simulink model "forced_choice"  (Simulink 8.5)
settings: Solver=FixedStepDiscrete  StartTime=0.0  StopTime=Inf  FixedStep=.001  RelTol=1e-3
libraries: limblab x14, slrtlib x2, IntelSMIlibR2007b x1
CloseFcn:
  | rtwprivate ssgencode ModelCloseRequest rwalk_multi_local_v1
settings Model: Creator=limblab  LastModifiedBy=limblab  ExtModeArmWhenConnect=off
settings SolverCC: EnableConcurrentExecution=on
settings DataIOCC: LimitDataPoints=off  SaveFormat=StructureWithTime  SaveState=on  SignalLoggingName=sigsOut
settings OptimizationCC: BlockReduction=off  BooleanDataType=off  OptimizeBlockIOStorage=off  BufferReuse=off  GlobalBufferReuse=off  ExpressionFolding=off  LocalBlockOutputs=off  InitFltsAndDblsToZero=on
settings DebuggingCC: SaveWithParameterizedLinksMsg=none  SignalResolutionControl=TryResolveAllWithWarning  MultiTaskDSMMsg=warning  MultiTaskCondExecSysMsg=none  FcnCallInpInsideContextMsg=UseLocalSettings
settings HardwareCC: ProdIntDivRoundTo=Zero  ProdEndianess=LittleEndian  ProdLongLongMode=on  ProdHWDeviceType=Generic->32-bit x86 compatible  TargetIntDivRoundTo=Floor  TargetEndianess=LittleEndian  TargetHWDeviceType=32-bit xPC Target (Intel Pentium)
settings SFSimCC: SimParseCustomCode=off
settings RTWCC: SystemTargetFile=slrt.tlc  TemplateMakefile=slrt_default_tmf  Description=Simulink Real-Time  GenerateReport=on  RTWCompilerOptimization=on
settings SimulinkRealTimeCC: TargetFcnLib=ansi_tfl_tmw.mat  GeneratePreprocessorConditionals=Disable all

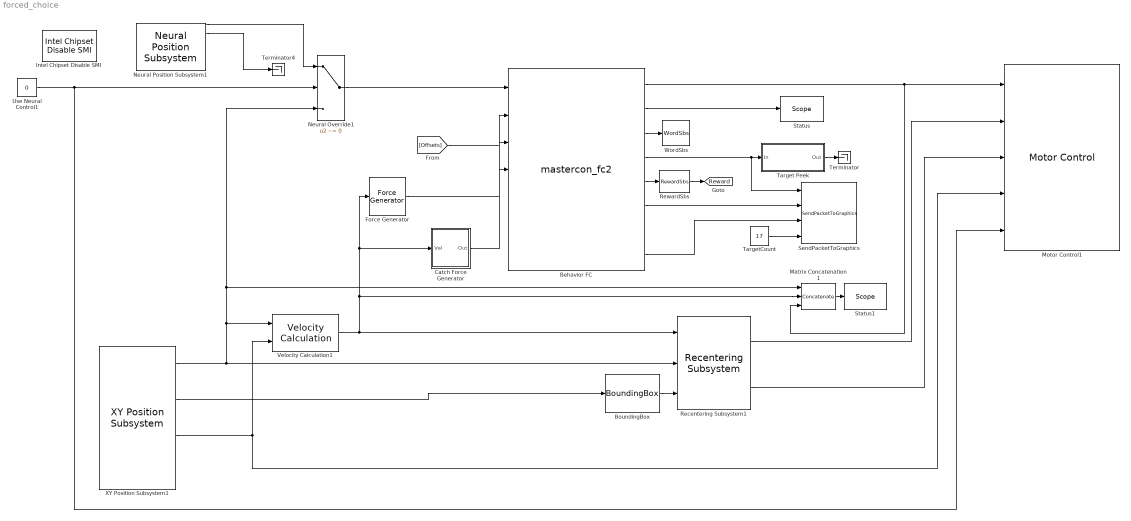
== system forced_choice ==
  Behavior FC : S-Function  FunctionName=mastercon_fc2  Parameters=0 0 3 8 0 0 0 1 0 0 2 .15 .2 .1 .3 .2 .7 .5 1 .2 1 1 1 0 16 .3 1 1
      mask Display:
      | disp('Master Control')
      | port_label('input',1,'pos')
      | port_label('input',2,'pos offsets')
      | port_label('input',3,'force')
      | port_label('input',4,'catch force')
      | port_label('output',1,'force')
      | port_label('output',2,'status')
      | port_label('output',3,'word')
      | port_label('output',4,'targets')
      | port_label('output',5,'reward')
      | port_label('output',6,'tone')
      | port_label('output',7,'version')
      | port_label('output',8,'pos')
  BoundingBox : limblab/BoundingBox
  Catch Force Generator : Subsystem
  Force Generator : limblab/Force Generator
  Intel Chipset Disable SMI : IntelSMIlibR2007b/Intel Chipset Disable SMI
  Matrix Concatenation1 : Concatenate  NumInputs=3
  Motor Control1 : limblab/Motor Control
  Neural Override1 : Switch  Criteria=u2 ~= 0  ZeroCross=off
  Neural Position Subsystem1 : limblab/Neural Position Subsystem
  Recentering Subsystem1 : limblab/Recentering Subsystem
  RewardSbs : limblab/RewardSbs
  SendPacketToGraphics : limblab/SendPacketToGraphics
  Status : slrtlib/Displays and Logging/Scope   scopeno=1  scopetype=Target  autostart=on  viewmode=Numerical  formatstr='%6.0f state,%6.0f rewards,%6.0f aborts,%6.0f fails,%6.0f incompl'  grid=on  ylimits=[-10,10]  nosamples=10  noprepostsamples=0  interleave=10  triggermode=FreeRun  triggersignal=1  trigsignalfromport=off  triggerlevel=0.0  triggerslope=Either  triggerscope=1  triggersample=0  filename=data.dat  mode=Lazy  writesize=512  autorestart=off  dynamicfilemode=off  maxwritefilesize=512*1024^2
  Status1 : slrtlib/Displays and Logging/Scope   scopeno=3  scopetype=Target  autostart=on  viewmode=Numerical  formatstr='%6.0f x,%6.0f y,%6.0f vx,%6.0f vy,%6.0f fx,%6.0f fy'  grid=on  ylimits=[-10,10]  nosamples=10  noprepostsamples=0  interleave=10  triggermode=FreeRun  triggersignal=1  trigsignalfromport=off  triggerlevel=0.0  triggerslope=Either  triggerscope=1  triggersample=0  filename=data.dat  mode=Lazy  writesize=512  autorestart=off  dynamicfilemode=off  maxwritefilesize=512*1024^2
  Target Peek : Subsystem
  TargetCount : Constant  Value=17
  Terminator : Terminator
  Terminator4 : Terminator
  Use Neural Control1 : Constant  Value=0
  Velocity Calculation1 : limblab/Velocity Calculation
  WordSbs : limblab/WordSbs
  XY Position Subsystem1 : limblab/XY Position Subsystem
  tag scope: Reward=global
  wires:
  Velocity Calculation1/1 -> Recentering Subsystem1/1, Force Generator/1, Catch Force Generator/1(Vel), Matrix Concatenation1/2
  XY Position Subsystem1/1 -> Neural Override1/3, Matrix Concatenation1/1, Velocity Calculation1/1, Recentering Subsystem1/2
  Behavior FC/2 -> Status/1
  Behavior FC/3 -> WordSbs/1
  Behavior FC/4 -> Target Peek/1(In), SendPacketToGraphics/1
  Behavior FC/5 -> RewardSbs/1
  BoundingBox/1 -> Recentering Subsystem1/3
  XY Position Subsystem1/3 -> Velocity Calculation1/2, Motor Control1/4
  XY Position Subsystem1/2 -> BoundingBox/1
  Recentering Subsystem1/2 -> Motor Control1/3
  Recentering Subsystem1/1 -> Motor Control1/2
  Behavior FC/8 -> SendPacketToGraphics/3
  Behavior FC/6 -> SendPacketToGraphics/2
  RewardSbs/1 -> [Reward]
  Use Neural Control1/1 -> Motor Control1/5, Neural Override1/2
  Neural Position Subsystem1/1 -> Neural Override1/1
  Neural Position Subsystem1/2 -> Terminator4/1
  Neural Override1/1 -> Behavior FC/1
  Target Peek/1(Out) -> Terminator/1
  TargetCount/1 -> SendPacketToGraphics/4
  Catch Force Generator/1(Out) -> Behavior FC/4
  Force Generator/1 -> Behavior FC/3
  [Offsets] -> Behavior FC/2
  Matrix Concatenation1/1 -> Status1/1
  Behavior FC/1 -> Matrix Concatenation1/3, Motor Control1/1

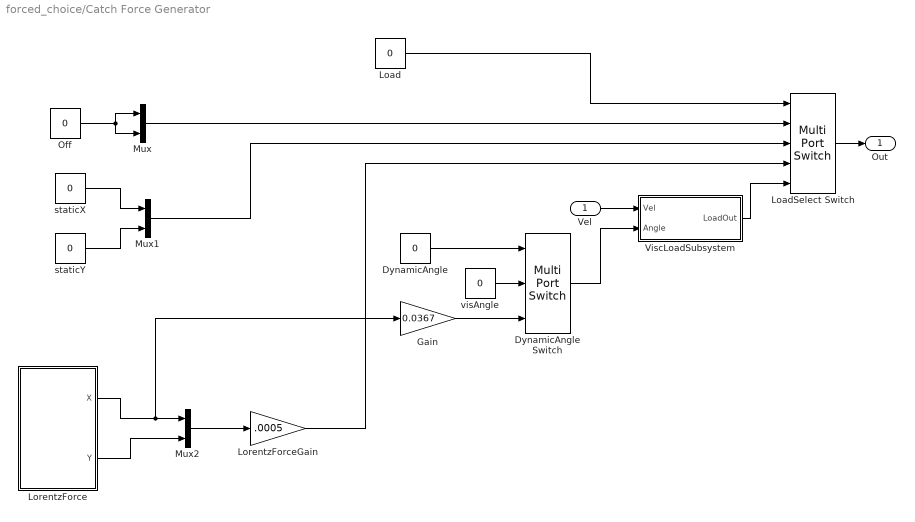
== system forced_choice/Catch Force Generator ==
  Vel : Inport
  DynamicAngle : Constant  Value=0
  DynamicAngle Switch : MultiPortSwitch  DataPortOrder=Zero-based contiguous  Inputs=2  zeroidx=on
  Gain : Gain  Gain=0.0367
  Load : Constant  Value=0
  LoadSelect Switch : MultiPortSwitch  DataPortOrder=Zero-based contiguous  Inputs=4  zeroidx=on
  LorentzForce : Subsystem
  LorentzForceGain : Gain  Gain=.0005
  Mux : Mux  Inputs=2
  Mux1 : Mux  Inputs=2
  Mux2 : Mux  Inputs=2
  Off : Constant  Value=0
  ViscLoadSubsystem : Subsystem
  staticX : Constant  Value=0
  staticY : Constant  Value=0
  visAngle : Constant  Value=0
  Out : Outport
  wires:
  Off/1 -> Mux/2, Mux/1
  LoadSelect Switch/1 -> Out/1
  Mux/1 -> LoadSelect Switch/2
  Load/1 -> LoadSelect Switch/1
  Mux1/1 -> LoadSelect Switch/3
  staticX/1 -> Mux1/1
  staticY/1 -> Mux1/2
  LorentzForce/1(X) -> Mux2/1, Gain/1
  LorentzForce/2(Y) -> Mux2/2
  Mux2/1 -> LorentzForceGain/1
  LorentzForceGain/1 -> LoadSelect Switch/4
  Vel/1 -> ViscLoadSubsystem/1(Vel)
  ViscLoadSubsystem/1(LoadOut) -> LoadSelect Switch/5
  visAngle/1 -> DynamicAngle Switch/2
  DynamicAngle/1 -> DynamicAngle Switch/1
  DynamicAngle Switch/1 -> ViscLoadSubsystem/2(Angle)
  Gain/1 -> DynamicAngle Switch/3

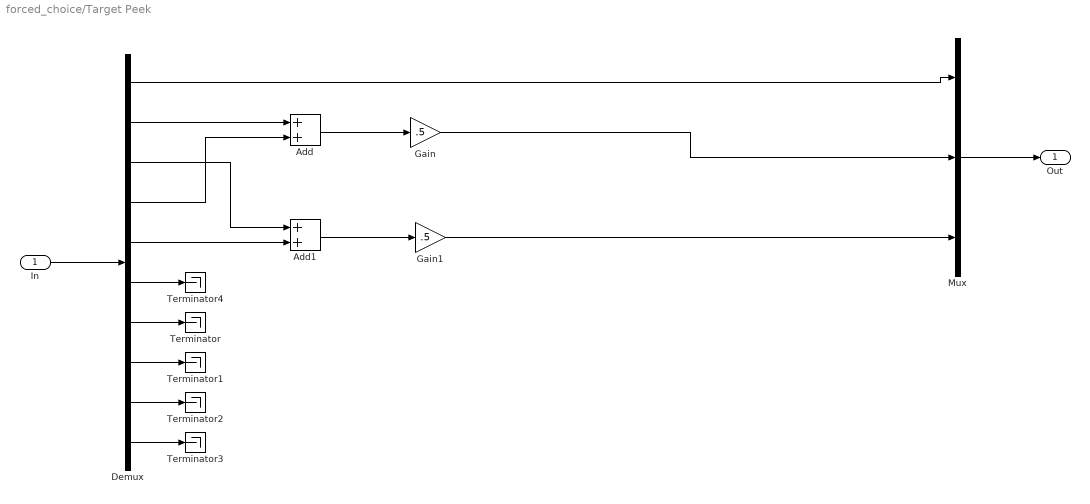
== system forced_choice/Target Peek ==
  In : Inport
  Add : Sum
  Add1 : Sum
  Demux : Demux  Outputs=10
  Gain : Gain  Gain=.5
  Gain1 : Gain  Gain=.5
  Mux : Mux  Inputs=3
  Terminator{,1..4} (5 alike) : Terminator
  Out : Outport
  wires:
  In/1 -> Demux/1
  Mux/1 -> Out/1
  Demux/1 -> Mux/1
  Add/1 -> Gain/1
  Add1/1 -> Gain1/1
  Gain1/1 -> Mux/3
  Demux/7 -> Terminator/1
  Demux/8 -> Terminator1/1
  Demux/9 -> Terminator2/1
  Demux/10 -> Terminator3/1
  Demux/2 -> Add/1
  Demux/4 -> Add/2
  Demux/3 -> Add1/1
  Demux/5 -> Add1/2
  Demux/6 -> Terminator4/1
  Gain/1 -> Mux/2

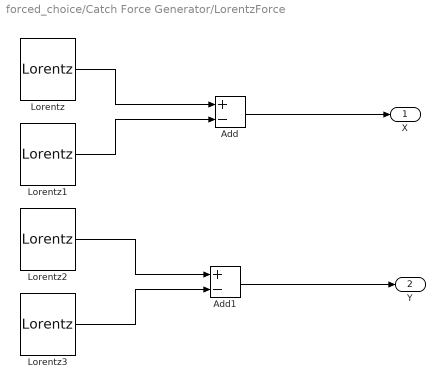
== system forced_choice/Catch Force Generator/LorentzForce ==
  Add : Sum  Inputs=+-
  Add1 : Sum  Inputs=+-
  Lorentz : limblab/Lorentz  y0=.1
  Lorentz1 : limblab/Lorentz  y0=.2
  Lorentz2 : limblab/Lorentz  y0=.3
  Lorentz3 : limblab/Lorentz  y0=.4
  X : Outport
  Y : Outport  Port=2
  wires:
  Lorentz/1 -> Add/1
  Lorentz1/1 -> Add/2
  Add/1 -> X/1
  Lorentz2/1 -> Add1/1
  Lorentz3/1 -> Add1/2
  Add1/1 -> Y/1

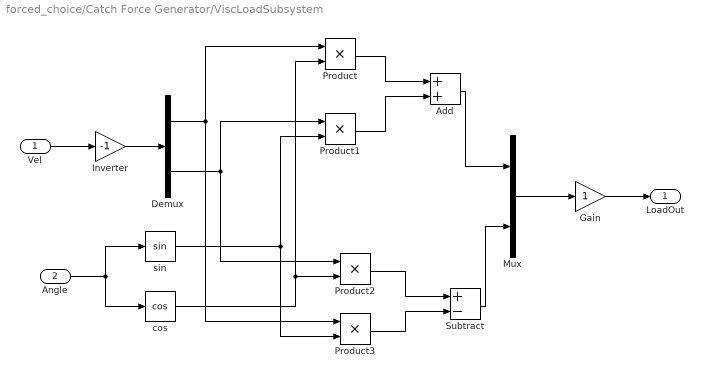
== system forced_choice/Catch Force Generator/ViscLoadSubsystem ==
  Vel : Inport
  Angle : Inport  Port=2
  Add : Sum
  Demux : Demux  Outputs=2
  Gain : Gain
  Inverter : Gain  Gain=-1
  Mux : Mux  Inputs=2
  Product{,1..3} (4 alike) : Product  RndMeth=Zero
  Subtract : Sum  Inputs=+-
  cos : Trigonometry  Operator=cos
  sin : Trigonometry
  LoadOut : Outport
  wires:
  Mux/1 -> Gain/1
  Gain/1 -> LoadOut/1
  Angle/1 -> sin/1, cos/1
  Add/1 -> Mux/1
  Subtract/1 -> Mux/2
  Product/1 -> Add/1
  Product1/1 -> Add/2
  Product2/1 -> Subtract/1
  Product3/1 -> Subtract/2
  Demux/1 -> Product/1, Product3/1
  cos/1 -> Product/2, Product2/2
  Demux/2 -> Product1/1, Product2/1
  sin/1 -> Product1/2, Product3/2
  Inverter/1 -> Demux/1
  Vel/1 -> Inverter/1
